simulink model "Task3Pro"  (R2023b)
settings: Solver=VariableStepAuto  StartTime=0.0  StopTime=10.0  RelTol=1e-3
libraries: simulink_extras x2
settings Model: Creator=danish  LastModifiedBy=danish

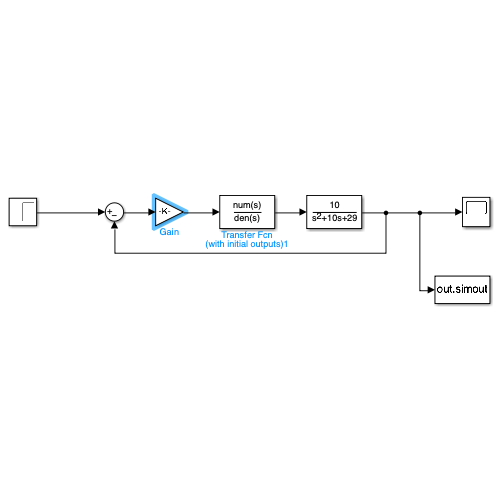
[thumbnail: Simulink's stored preview of the top-level diagram]
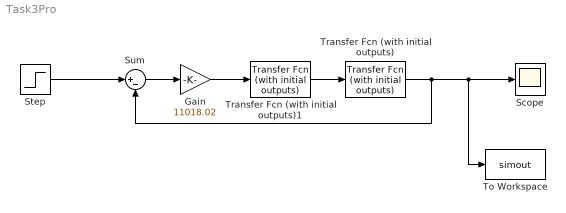
== system Task3Pro ==
  Gain : Gain  Gain=11018.02
  Scope : Scope
  Step : Step  SampleTime=0
  Sum : Sum  Inputs=|+-
  To Workspace : ToWorkspace  VariableName=simout  SaveFormat=Timeseries  SampleTime=-1
  Transfer Fcn (with initial outputs) : simulink_extras/Additional Linear/Transfer Fcn (with initial outputs)  N=[10]  D=[1 10 29]  Y0=.5  U0=0
  Transfer Fcn (with initial outputs)1 : simulink_extras/Additional Linear/Transfer Fcn (with initial outputs)  N=[1 6.01 0.06]  D=[1 120 2000 0]  Y0=.5  U0=0
  wires:
  Step/1 -> Sum/1
  Transfer Fcn (with initial outputs)1/1 -> Transfer Fcn (with initial outputs)/1
  Gain/1 -> Transfer Fcn (with initial outputs)1/1
  Sum/1 -> Gain/1
  Transfer Fcn (with initial outputs)/1 -> Sum/2, To Workspace/1, Scope/1
